simulink model "FinalControl"  (R2020a)
settings: Solver=VariableStepAuto  StartTime=0.0  StopTime=10.0  RelTol=1e-3
settings Model: Creator=Joseph  LastModifiedBy=Joseph

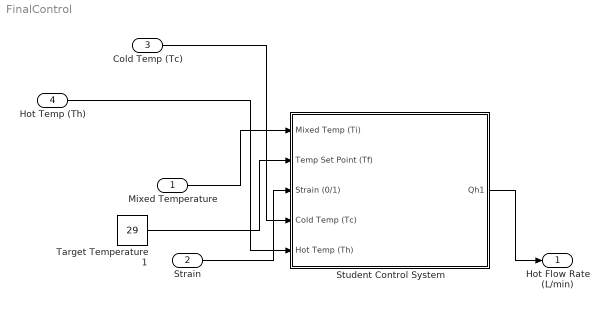
== system FinalControl ==
  Mixed Temperature : Inport
  Strain : Inport  Port=2
  Cold Temp (Tc) : Inport  Port=3
  Hot Temp (Th) : Inport  Port=4
  Student Control System : Subsystem
  Target Temperature 1 : Constant  Value=29
  Hot Flow Rate (L/min) : Outport
  wires:
  Target Temperature 1/1 -> Student Control System/2(Temp Set Point (Tf))
  Student Control System/1(Qh1) -> Hot Flow Rate (L/min)/1
  Mixed Temperature/1 -> Student Control System/1(Mixed Temp (Ti))
  Strain/1 -> Student Control System/3(Strain (0/1))
  Cold Temp (Tc)/1 -> Student Control System/4(Cold Temp (Tc))
  Hot Temp (Th)/1 -> Student Control System/5(Hot Temp (Th))

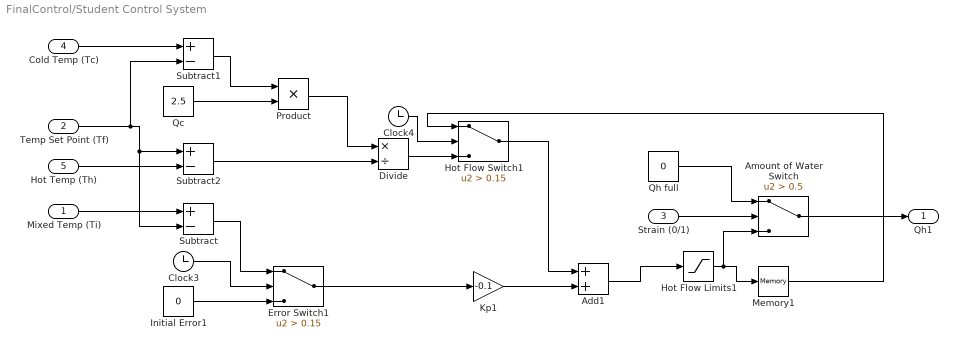
== system FinalControl/Student Control System ==
  Mixed Temp (Ti) : Inport
  Temp Set Point (Tf) : Inport  Port=2
  Strain (0/1) : Inport  Port=3
  Cold Temp (Tc) : Inport  Port=4
  Hot Temp (Th) : Inport  Port=5
  Add1 : Sum
  Amount of Water Switch : Switch  Criteria=u2 > Threshold  Threshold=0.5
  Clock3 : Clock
  Clock4 : Clock
  Divide : Product  Inputs=*/
  Error Switch1 : Switch  Criteria=u2 > Threshold  Threshold=0.15
  Hot Flow Limits1 : Saturate  UpperLimit=3.5  LowerLimit=1.5
  Hot Flow Switch1 : Switch  Criteria=u2 > Threshold  Threshold=0.15
  Initial Error1 : Constant  Value=0
  Kp1 : Gain  Gain=-0.1
  Memory1 : Memory
  Product : Product
  Qc : Constant  Value=2.5
  Qh full : Constant  Value=0
  Subtract : Sum  Inputs=+-
  Subtract1 : Sum  Inputs=+-
  Subtract2 : Sum  Inputs=+-
  Qh1 : Outport
  wires:
  Amount of Water Switch/1 -> Qh1/1
  Memory1/1 -> Hot Flow Switch1/1
  Subtract2/1 -> Divide/2
  Strain (0/1)/1 -> Amount of Water Switch/2
  Product/1 -> Divide/1
  Cold Temp (Tc)/1 -> Subtract1/1
  Hot Temp (Th)/1 -> Subtract2/2
  Subtract1/1 -> Product/1
  Qc/1 -> Product/2
  Qh full/1 -> Amount of Water Switch/1
  Temp Set Point (Tf)/1 -> Subtract2/1, Subtract/2, Subtract1/2
  Clock4/1 -> Hot Flow Switch1/2
  Subtract/1 -> Error Switch1/1
  Initial Error1/1 -> Error Switch1/3
  Error Switch1/1 -> Kp1/1
  Clock3/1 -> Error Switch1/2
  Mixed Temp (Ti)/1 -> Subtract/1
  Kp1/1 -> Add1/2
  Hot Flow Switch1/1 -> Add1/1
  Add1/1 -> Hot Flow Limits1/1
  Divide/1 -> Hot Flow Switch1/3
  Hot Flow Limits1/1 -> Memory1/1, Amount of Water Switch/3
